simulink model "Trajectory_Tracking_Simulink"  (R2019a)
settings: Solver=VariableStepAuto  StartTime=0.0  StopTime=35  RelTol=1e-3
InitFcn:
  | current_path = pwd;
  | root_folder = strfind(current_path, 'Trajectory_Tracking_Simulation');
  | root_path = current_path( 1 : ( root_folder + 29 ) );
  | initial_folder_path = string(root_path) + '/Initial';
  | addpath(initial_folder_path);
  | run('Initial_Script.m');
model workspace (MAT data in the model file):
  object = [3707764736; 2; 1; 1; 1; 1]
libraries: vrlib x2
settings Model: OrderedModelArguments=off  Creator=Admin  LastModifiedBy=Admin

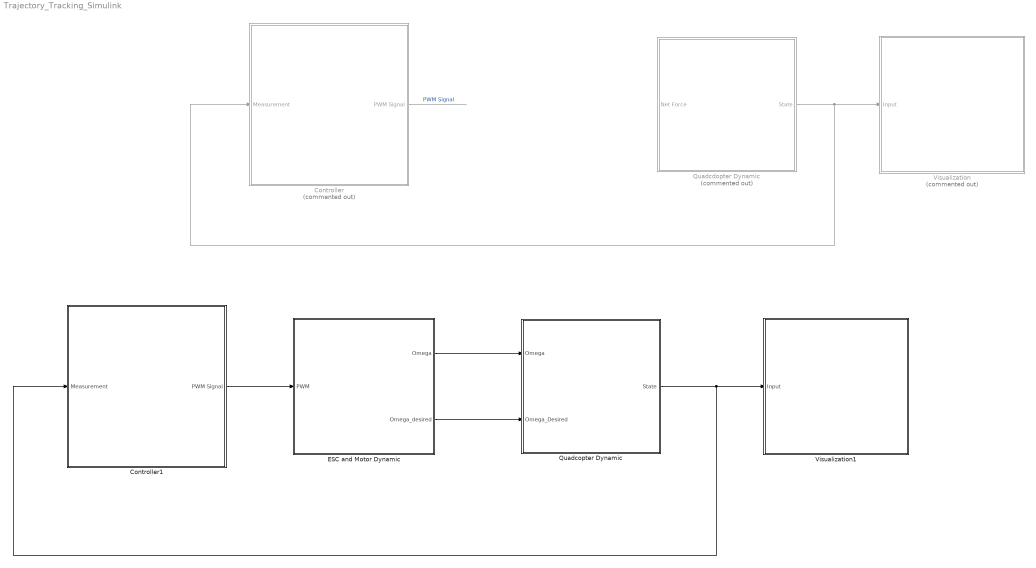
== system Trajectory_Tracking_Simulink ==
  Controller : Subsystem  Commented=on
      mask Display: image('PX4_Picture.jpg');
  Controller1 : Subsystem
      mask Display: image('PX4_Picture.jpg');
  ESC and Motor Dynamic : Subsystem  mask{ct=3.677609694514498e-06, cq=3.677609694514498e-06 / 12, alpha=23 * 1e-3}
      mask prompts: ct "Thrust Coefficent"; cq "Torque Coefficent"; alpha "Delay Time"
      mask DialogControl DescGroupVar Prompt: ESC and Motor Dynamic
      mask DialogControl DescTextVar Prompt: This bock describe ESC and Motor Dynamic
      mask Display: image('ESC_Picture.jpg');
  Quadcdopter Dynamic : Subsystem  Commented=on
      mask Display: image('Kinematic_Diagram.jpg');
  Quadcopter Dynamic : Subsystem
      mask Display: image('Kinematic_Diagram.jpg');
  Visualization : Subsystem  Commented=on
      mask Display: image('VR_Picture.jpg');
  Visualization1 : Subsystem
      mask Display: image('VR_Picture.jpg');
  wires:
  Quadcdopter Dynamic/1("State ") -> Controller/1("Measurement "), Visualization/1("Input ")
  Controller/1(PWM Signal) -> ?  "PWM Signal"
  ? -> Quadcdopter Dynamic/1("Net Force ")  "Force"
  Controller1/1(PWM Signal) -> ESC and Motor Dynamic/1(PWM)
  ESC and Motor Dynamic/1(Omega) -> Quadcopter Dynamic/1("Omega ")
  ESC and Motor Dynamic/2(Omega_desired) -> Quadcopter Dynamic/2(Omega_Desired)
  Quadcopter Dynamic/1("State ") -> Controller1/1("Measurement "), Visualization1/1("Input ")

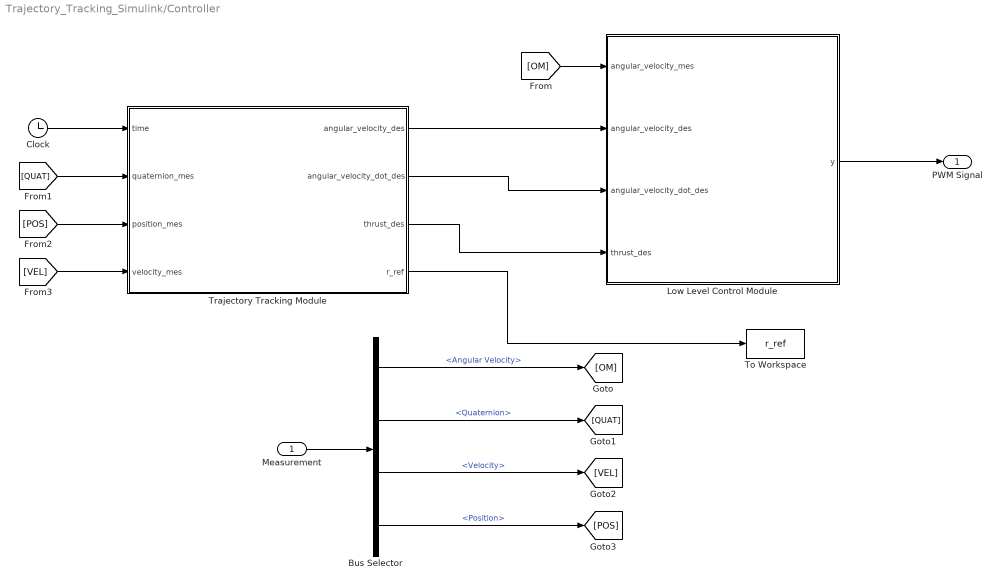
== system Trajectory_Tracking_Simulink/Controller ==
  "Measurement " : Inport
  Bus Selector : BusSelector  OutputSignals=Angular Velocity,Quaternion,Velocity,Position
  Clock : Clock
  Low Level Control Module : MATLAB Function  TreatAsAtomicUnit=on
  To Workspace : ToWorkspace  VariableName=r_ref  SaveFormat=Timeseries  SampleTime=-1
  Trajectory Tracking Module : MATLAB Function  TreatAsAtomicUnit=on
  PWM Signal : Outport
  wires:
  "Measurement "/1 -> Bus Selector/1
  Low Level Control Module/1(y) -> PWM Signal/1
  Bus Selector/1 -> [OM]  "<Angular Velocity>"
  [OM] -> Low Level Control Module/1(angular_velocity_mes)
  Bus Selector/2 -> [QUAT]  "<Quaternion>"
  Bus Selector/3 -> [VEL]  "<Velocity>"
  [QUAT] -> Trajectory Tracking Module/2(quaternion_mes)
  [POS] -> Trajectory Tracking Module/3(position_mes)
  [VEL] -> Trajectory Tracking Module/4(velocity_mes)
  Clock/1 -> Trajectory Tracking Module/1(time)
  Bus Selector/4 -> [POS]  "<Position>"
  Trajectory Tracking Module/1(angular_velocity_des) -> Low Level Control Module/2(angular_velocity_des)
  Trajectory Tracking Module/2(angular_velocity_dot_des) -> Low Level Control Module/3(angular_velocity_dot_des)
  Trajectory Tracking Module/3(thrust_des) -> Low Level Control Module/4(thrust_des)
  Trajectory Tracking Module/4(r_ref) -> To Workspace/1

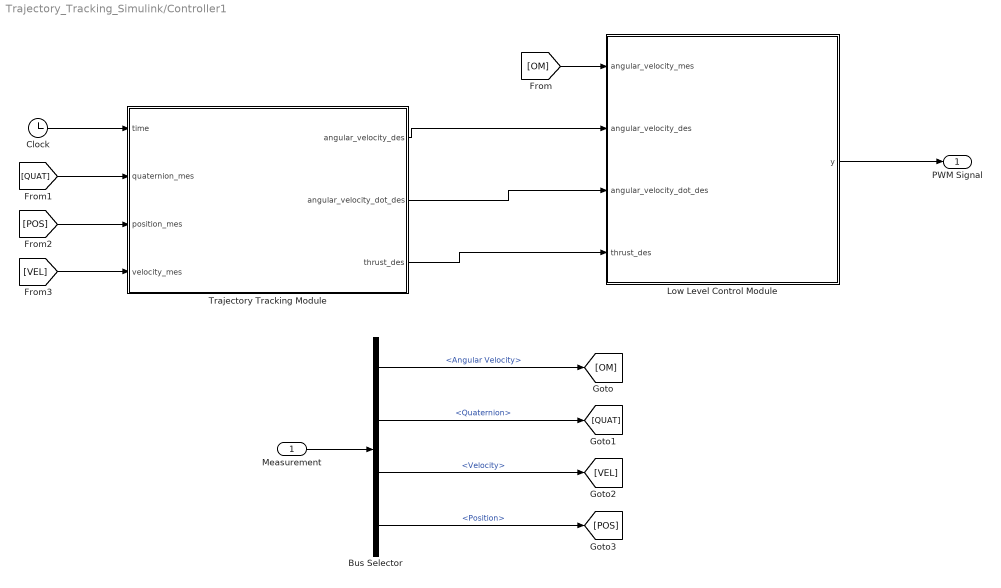
== system Trajectory_Tracking_Simulink/Controller1 ==
  "Measurement " : Inport
  Bus Selector : BusSelector  OutputSignals=Angular Velocity,Quaternion,Velocity,Position
  Clock : Clock
  Low Level Control Module : MATLAB Function  TreatAsAtomicUnit=on
  Trajectory Tracking Module : MATLAB Function  TreatAsAtomicUnit=on
  PWM Signal : Outport
  wires:
  "Measurement "/1 -> Bus Selector/1
  Low Level Control Module/1(y) -> PWM Signal/1
  Bus Selector/1 -> [OM]  "<Angular Velocity>"
  [OM] -> Low Level Control Module/1(angular_velocity_mes)
  Bus Selector/2 -> [QUAT]  "<Quaternion>"
  Bus Selector/3 -> [VEL]  "<Velocity>"
  [QUAT] -> Trajectory Tracking Module/2(quaternion_mes)
  [POS] -> Trajectory Tracking Module/3(position_mes)
  [VEL] -> Trajectory Tracking Module/4(velocity_mes)
  Clock/1 -> Trajectory Tracking Module/1(time)
  Bus Selector/4 -> [POS]  "<Position>"
  Trajectory Tracking Module/1(angular_velocity_des) -> Low Level Control Module/2(angular_velocity_des)
  Trajectory Tracking Module/2(angular_velocity_dot_des) -> Low Level Control Module/3(angular_velocity_dot_des)
  Trajectory Tracking Module/3(thrust_des) -> Low Level Control Module/4(thrust_des)

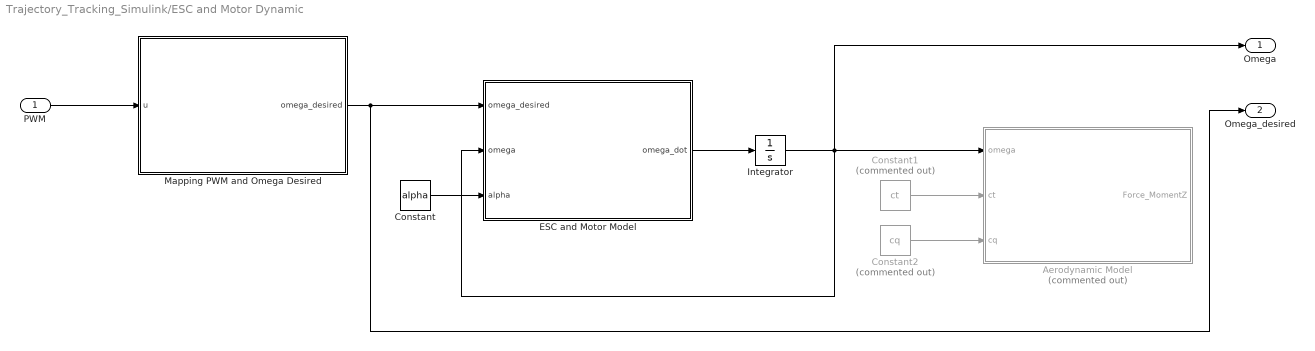
== system Trajectory_Tracking_Simulink/ESC and Motor Dynamic ==
  PWM : Inport
  Aerodynamic Model : MATLAB Function  Commented=on  TreatAsAtomicUnit=on  mask{ct=ct, cq=cq}
      mask prompts: ct "Thrust Coefficent"; cq "Torque Coefficent"
  Constant : Constant  Value=alpha
  Constant1 : Constant  Commented=on  Value=ct
  Constant2 : Constant  Commented=on  Value=cq
  ESC and Motor Model : MATLAB Function  TreatAsAtomicUnit=on  mask{alpha=alpha}
      mask prompts: alpha "Delay Time"
  Integrator : Integrator  InitialCondition=516.5 * ones(4,1)
  Mapping PWM and Omega Desired : MATLAB Function  TreatAsAtomicUnit=on
  Omega : Outport
  Omega_desired : Outport  Port=2
  wires:
  ESC and Motor Model/1(omega_dot) -> Integrator/1
  Integrator/1 -> Omega/1, Aerodynamic Model/1(omega), ESC and Motor Model/2(omega)
  PWM/1 -> Mapping PWM and Omega Desired/1(u)
  Constant/1 -> ESC and Motor Model/3(alpha)
  Constant1/1 -> Aerodynamic Model/2(ct)
  Constant2/1 -> Aerodynamic Model/3(cq)
  Mapping PWM and Omega Desired/1(omega_desired) -> ESC and Motor Model/1(omega_desired), Omega_desired/1

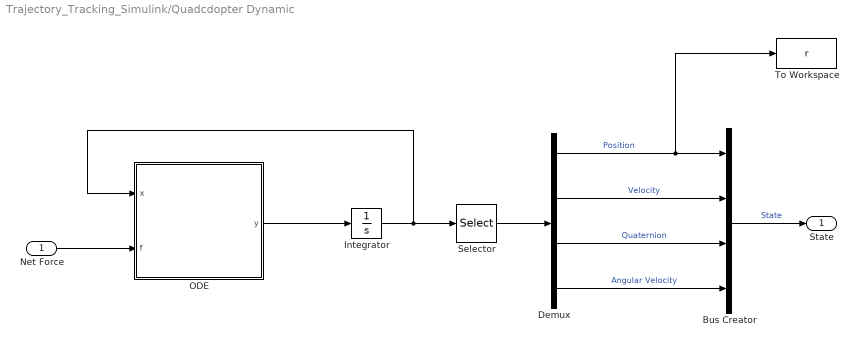
== system Trajectory_Tracking_Simulink/Quadcdopter Dynamic ==
  "Net Force " : Inport
  Bus Creator : BusCreator  Inputs=4
  Demux : Demux  Outputs=[3 3 4 3]
  Integrator : Integrator  InitialCondition=[zeros(3,1); zeros(3,1); [1; 0; 0; 0]; [0; 0; 0]]
  ODE : MATLAB Function  TreatAsAtomicUnit=on
  Selector : Selector  InputPortWidth=13  IndexOptions=Select all  Indices=1  OutputSizes=1
  To Workspace : ToWorkspace  VariableName=r  SaveFormat=Timeseries  SampleTime=-1
  "State " : Outport
  wires:
  Integrator/1 -> Selector/1, ODE/1(x)
  Selector/1 -> Demux/1
  ODE/1(y) -> Integrator/1
  Demux/4 -> Bus Creator/4  "Angular Velocity"
  "Net Force "/1 -> ODE/2(f)
  Demux/1 -> To Workspace/1, Bus Creator/1  "Position"
  Demux/2 -> Bus Creator/2  "Velocity"
  Demux/3 -> Bus Creator/3  "Quaternion"
  Bus Creator/1 -> "State "/1  "State"

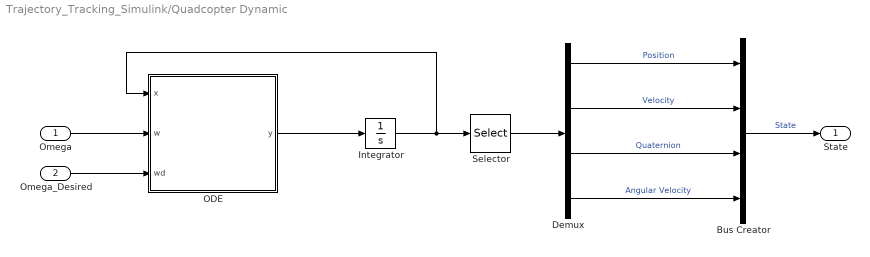
== system Trajectory_Tracking_Simulink/Quadcopter Dynamic ==
  "Omega " : Inport
  Omega_Desired : Inport  Port=2
  Bus Creator : BusCreator  Inputs=4
  Demux : Demux  Outputs=[3 3 4 3]
  Integrator : Integrator  InitialCondition=[zeros(3,1); zeros(3,1); [1; 0;0 ;0]; [0; 0; 0]]
  ODE : MATLAB Function  TreatAsAtomicUnit=on
  Selector : Selector  InputPortWidth=13  IndexOptions=Select all  Indices=1  OutputSizes=1
  "State " : Outport
  wires:
  Integrator/1 -> ODE/1(x), Selector/1
  Selector/1 -> Demux/1
  ODE/1(y) -> Integrator/1
  Demux/4 -> Bus Creator/4  "Angular Velocity"
  "Omega "/1 -> ODE/2(w)
  Demux/1 -> Bus Creator/1  "Position"
  Demux/2 -> Bus Creator/2  "Velocity"
  Demux/3 -> Bus Creator/3  "Quaternion"
  Bus Creator/1 -> "State "/1  "State"
  Omega_Desired/1 -> ODE/3(wd)

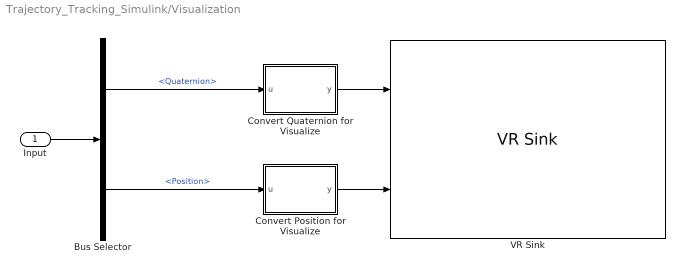
== system Trajectory_Tracking_Simulink/Visualization ==
  "Input " : Inport
  Bus Selector : BusSelector  OutputSignals=Quaternion,Position
  "Convert Position for Visualize " : MATLAB Function  TreatAsAtomicUnit=on
  "Convert Quaternion for Visualize " : MATLAB Function  TreatAsAtomicUnit=on
  VR Sink : vrlib/VR Sink  InstantiateOnLoad=on  SampleTime=0.01  ViewEnable=on  RemoteChange=off  RemoteView=off  FieldsWritten=FBX_Quadcopter_3d_Model_Transform.rotation.4.1.1.double#FBX_Quadcopter_3d_Model_Transform.translation.3.1.1.double  WorldFileName=3d_Model.wrl  AutoView=off  VideoDimensions=[]  AllowVariableSize=off
      settings: SourceProductName=Simulink
  wires:
  "Convert Quaternion for Visualize "/1(y) -> VR Sink/1
  "Convert Position for Visualize "/1(y) -> VR Sink/2
  "Input "/1 -> Bus Selector/1
  Bus Selector/1 -> "Convert Quaternion for Visualize "/1(u)  "<Quaternion>"
  Bus Selector/2 -> "Convert Position for Visualize "/1(u)  "<Position>"

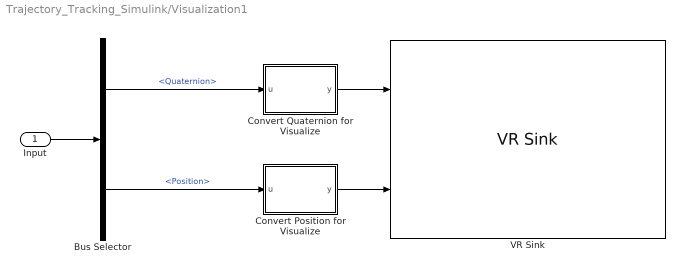
== system Trajectory_Tracking_Simulink/Visualization1 ==
  "Input " : Inport
  Bus Selector : BusSelector  OutputSignals=Quaternion,Position
  "Convert Position for Visualize " : MATLAB Function  TreatAsAtomicUnit=on
  "Convert Quaternion for Visualize " : MATLAB Function  TreatAsAtomicUnit=on
  VR Sink : vrlib/VR Sink  InstantiateOnLoad=on  SampleTime=0.01  ViewEnable=on  RemoteChange=off  RemoteView=off  FieldsWritten=FBX_Quadcopter_3d_Model_Transform.rotation.4.1.1.double#FBX_Quadcopter_3d_Model_Transform.translation.3.1.1.double  WorldFileName=3d_Model.wrl  AutoView=off  VideoDimensions=[]  AllowVariableSize=off  FigureProperties="{'Position', 'Name', 'Viewpoint', 'CameraBound', 'CameraDirection', 'CameraPosition', 'CameraUpVector', 'ZoomFactor', 'Antialiasing', 'Headlight', 'Lighting', 'NavPanel', 'Sound', 'StatusBar', 'Stereo3D', 'Stereo3DCameraOffset', 'Stereo3DHIT', 'ToolBar', 'Textures', 'Transparency', 'Triad', 'Wireframe', 'NavZones', 'NavMode', 'NavSpeed', 'CaptureFileFormat', 'CaptureFileName', 'Record2DCompressMethod', 'Record2DCompressQuality', 'Record2D', 'Record2DFileName', 'Record2DFPS'; [1.0000000000000000e+00   7.6000000000000000e+01   1.9200000000000000e+03   9.5300000000000000e+02], '', 'Perspective View', 'on', [0.0000000000000000e+00   0.0000000000000000e+00  -1.0000000000000000e+00], [0.0000000000000000e+00   0.0000000000000000e+00   0.0000000000000000e+00], [0.0000000000000000e+00   1.0000000000000000e+00   0.0000000000000000e+00], [3.7974983358324148e+00], 'on', 'on', 'on', 'halfbar', 'on', 'on', 'off', [1.0000000149011612e-01], [0.0000000000000000e+00], 'on', 'on', 'on', 'none', 'off', 'off', 'fly', 'normal', 'tif', '%f_anim_%n.tif', 'auto', [7.5000000000000000e+01], 'off', '%f_anim_%n.avi', 'auto'}"
      settings: SourceProductName=Simulink
  wires:
  "Convert Quaternion for Visualize "/1(y) -> VR Sink/1
  "Convert Position for Visualize "/1(y) -> VR Sink/2
  "Input "/1 -> Bus Selector/1
  Bus Selector/1 -> "Convert Quaternion for Visualize "/1(u)  "<Quaternion>"
  Bus Selector/2 -> "Convert Position for Visualize "/1(u)  "<Position>"

== matlab function Trajectory_Tracking_Simulink/Quadcdopter Dynamic/ODE ==
  settings: updateMethod=CONTINUOUS
  data: x input; y output; f input
function y = fcn(x, f)
%%
m = 1.18;
g = [0; 0; -9.81];
a = 0.255/2;
k = 0.0174;
Ixx = 0.0144;
Iyy = 0.0145;
Izz = 0.0156;
J = diag([Ixx, Iyy, Izz]);

%%
r = x(1:3);
v = x(4:6);
q = x(7:10);
omega = x(11:13);

%%
torque = [a, -a, -a, a; -a, -a, a, a; k, -k, k, -k] * f;  
c_body_frame = [0, 0, 0, (1/m) * sum(f)];
c_world_frame = quatmultiply(quatmultiply(q', c_body_frame), quatconj(q'))';
OMEGA = 0.5 * [0, -omega'; omega, -skew(omega)];
x_dot = zeros(13,1);
x_dot(1:3) = v;
x_dot(4:6) = g + c_world_frame(2:end);
x_dot(7:10) = OMEGA * q;
x_dot(11:13) = J \ (torque - cross(omega, J * omega));

%%
y = x_dot;
end

== matlab function Trajectory_Tracking_Simulink/Controller/Low Level Control Module ==
  settings: updateMethod=DISCRETE  sampleTime=1/200
  data: angular_velocity_mes input; angular_velocity_des input; y output; angular_velocity_dot_des input; thrust_des input
function y = fcn(angular_velocity_mes, angular_velocity_des, angular_velocity_dot_des, thrust_des)
    persistent mixer omega_controller
    if isempty(mixer) 
        mixer = Mixer();
    end
    
    if isempty(omega_controller)
        omega_controller = AngularVelocityController();
    end
    
    omega_controller.updateAngularVelocityDesired(angular_velocity_des, angular_velocity_dot_des);
    omega_controller.updateTorqueDesired(angular_velocity_mes);
    
    
    mixer.setThrustTorqueSetpoint(omega_controller.torque_des, thrust_des);
    mixer.computeControlSignal();
    
    y = mixer.control_signal;
end

== matlab function Trajectory_Tracking_Simulink/Quadcopter Dynamic/ODE ==
  settings: updateMethod=CONTINUOUS
  data: x input; y output; w input; wd input
function y = fcn(x, w, wd)
%%
m = 1.18; % vehicle's mass
g = [0; 0; -9.81]; % gravity vector
a = 0.255/2; % half arm lenght
Ixx = 0.0257; % 
Iyy = 0.0255; %
Izz = 0.0321; %
Io = diag([Ixx, Iyy, Izz]); % vehicle's moment inertia
Ir = 8.67 * 1e-5; % rotor blade moment inertial
ct = 3.677609694514498e-06; % thrust coefficent
cq = ct / 12; % moment coefficient
rc = [7 * 1e-2; 6 * 1e-2; 0]; % center of mass in body frame
rc = [0;0;0];
alpha = 23 * 1e-3; % time delay of ESC + MOTOR + BLADE
%%
r = x(1:3);
v = x(4:6);
q = x(7:10);
W = x(11:13);

%% 
r_dot = v;

q_dot = 0.5 * quatmultiply( q', [0, W'] )';

G = [a*ct, -a*ct,  -a*ct, a*ct;
    -a*ct,  -a*ct, a*ct,  a*ct;
       cq,   -cq,    cq,   -cq;];
C0 = ct * skew(rc) * [zeros(2,4); ones(1,4)];
C1 = (1/alpha) * [zeros(2,4); -1, 1, -1, 1];
C2 = [0, 1, 0; -1, 0, 0; 0, 0, 0];
C3 = [-1 1 -1 1];
tau_g = Ir * ( C1 * (wd - w) + C2 * W * C3 * w );
tau_g = [0;0;0];
W_dot = (Io + m * skew(rc) * skew(rc)) \ ( (G - C0) * w.^2 - tau_g - cross( W, ( Io + m * (rc * rc')) * W ) );

Rz = [2 * (q(1) * q(3) + q(2) * q(4)); 2 * (q(3) * q(4) - q(1) * q(2)); 2 * (q(1)^2 +  q(4)^2) - 1] ;
F = m * g +  ct * Rz * [1 1 1 1] * w.^2;
term_1 = quatmultiply(quatmultiply(q', [0, cross(W_dot, rc)']), quatconj(q'));
term_2 = quatmultiply(quatmultiply(q', [0, (W' * W) * rc']), quatconj(q'));
v_dot = F/m - term_1(2:end)' + term_2(2:end)';

%%
x_dot = [r_dot; 
         v_dot; 
         q_dot;
         W_dot];
%%
y = x_dot;
end

== matlab function Trajectory_Tracking_Simulink/Visualization/Convert Position for Visualize  ==
  data: u input; y output
function y = fcn(u)
temp = quatmultiply(quatmultiply([0.5, -0.5, 0.5, 0.5], [0, u']), [0.5, 0.5, -0.5, -0.5]);
y = temp(2:end);

== matlab function Trajectory_Tracking_Simulink/Visualization/Convert Quaternion for Visualize  ==
  data: u input; y output
function y = fcn(u)
u = u./norm(u);
rotation_angle = 2 * acos(u(1));
rotation_axis = u(2:end)./(sin(0.5 * rotation_angle));
y = [0, -1, 0, 0; 0, 0, 1, 0; -1, 0, 0, 0; 0, 0, 0, 1]*[rotation_axis; rotation_angle];

== matlab function Trajectory_Tracking_Simulink/Controller/Trajectory Tracking Module ==
  settings: updateMethod=DISCRETE  sampleTime=1/50
  data: time input; quaternion_mes input; position_mes input; angular_velocity_des output; angular_velocity_dot_des output; thrust_des output; velocity_mes input; r_ref output
function [angular_velocity_des, angular_velocity_dot_des, thrust_des, r_ref] = fcn(time, quaternion_mes, position_mes, velocity_mes)
    persistent observer position_controller attitude_controller generator
    if isempty(observer)
        observer = GeneralObserver();
        observer.getInitMeasurement(quaternion_mes, position_mes);
        observer.init_time = time;
    end
    
    if isempty(position_controller)
        position_controller = PositionController();
    end
    
    if isempty(attitude_controller)
        attitude_controller = AttitudeController();
    end    
    
    if isempty(generator)
        generator = TrajectoryGenerator();
    end      

 
    observer.adjustMeasurement(quaternion_mes, position_mes, velocity_mes);
    observer.current_time = time;
    generator.updateTrajectorieStates(observer);
    
    position_controller.updateAcceleration(generator, observer);
    observer.computeQuadError(position_controller.acceleration_des, generator.phi);
	position_controller.updateAngularRef(generator , observer);

	attitude_controller.updateAngularVelocityDesired(observer, position_controller);
    
    angular_velocity_des = attitude_controller.omega_des;
    angular_velocity_dot_des = position_controller.omega_dot_ref;
    thrust_des = observer.c_des;
    
    r_ref = generator.r_ref;
    
end

== matlab function Trajectory_Tracking_Simulink/ESC and Motor Dynamic/Aerodynamic Model ==
  settings: updateMethod=CONTINUOUS
  data: omega input; Force_MomentZ output; ct input; cq input
function Force_MomentZ = fcn(omega, ct, cq)
% ct = 3.677609694514498e-06;
% cq = ct / 1.5;
Force_MomentZ = [ct * omega.^2; cq * omega.^2];           
end

== matlab function Trajectory_Tracking_Simulink/ESC and Motor Dynamic/ESC and Motor Model ==
  settings: updateMethod=CONTINUOUS
  data: omega_desired input; omega_dot output; omega input; alpha input
function omega_dot = fcn(omega_desired, omega, alpha)
% alpha = 23 * 1e-3;
omega_dot = (1 / alpha) * (omega_desired - omega);             
end

== matlab function Trajectory_Tracking_Simulink/ESC and Motor Dynamic/Mapping PWM and Omega Desired ==
  settings: updateMethod=CONTINUOUS
  data: u input; omega_desired output
function omega_desired = fcn(u)
omega_d_max = 1701;
omega_d_min = 516.5;
omega_desired = (omega_d_max - omega_d_min) * u + omega_d_min;
end

== matlab function Trajectory_Tracking_Simulink/Visualization1/Convert Position for Visualize  ==
  data: u input; y output
function y = fcn(u)
temp = quatmultiply(quatmultiply([0.5, -0.5, 0.5, 0.5], [0, u']), [0.5, 0.5, -0.5, -0.5]);
y = temp(2:end);

== matlab function Trajectory_Tracking_Simulink/Visualization1/Convert Quaternion for Visualize  ==
  data: u input; y output
function y = fcn(u)
u = u./norm(u);
rotation_angle = 2 * acos(u(1));
rotation_axis = u(2:end)./(sin(0.5 * rotation_angle));
y = [0, -1, 0, 0; 0, 0, 1, 0; -1, 0, 0, 0; 0, 0, 0, 1]*[rotation_axis; rotation_angle];

== matlab function Trajectory_Tracking_Simulink/Controller1/Low Level Control Module ==
  settings: updateMethod=DISCRETE  sampleTime=1/200
  data: angular_velocity_mes input; angular_velocity_des input; y output; angular_velocity_dot_des input; thrust_des input
function y = fcn(angular_velocity_mes, angular_velocity_des, angular_velocity_dot_des, thrust_des)
    persistent mixer omega_controller
    if isempty(mixer) 
        mixer = Mixer();
    end
    
    if isempty(omega_controller)
        omega_controller = AngularVelocityController();
    end
    
    omega_controller.updateAngularVelocityDesired(angular_velocity_des, angular_velocity_dot_des);
    omega_controller.updateTorqueDesired(angular_velocity_mes);
    
    
    mixer.setThrustTorqueSetpoint(omega_controller.torque_des, thrust_des);
    mixer.computeControlSignal();
    
    y = mixer.control_signal;
end

== matlab function Trajectory_Tracking_Simulink/Controller1/Trajectory Tracking Module ==
  settings: updateMethod=DISCRETE  sampleTime=1/50
  data: time input; quaternion_mes input; position_mes input; angular_velocity_des output; angular_velocity_dot_des output; thrust_des output; velocity_mes input
function [angular_velocity_des, angular_velocity_dot_des, thrust_des] = fcn(time, quaternion_mes, position_mes, velocity_mes)
    persistent observer position_controller attitude_controller generator
    if isempty(observer)
        observer = GeneralObserver();
        observer.getInitMeasurement(quaternion_mes, position_mes);
        observer.init_time = time;
    end
    
    if isempty(position_controller)
        position_controller = PositionController();
    end
    
    if isempty(attitude_controller)
        attitude_controller = AttitudeController();
    end    
    
    if isempty(generator)
        generator = TrajectoryGenerator();
    end      

 
    observer.adjustMeasurement(quaternion_mes, position_mes, velocity_mes);
    observer.current_time = time;
    generator.updateTrajectorieStates(observer);
    
    position_controller.updateAcceleration(generator, observer);
    observer.computeQuadError(position_controller.acceleration_des, generator.phi);
	position_controller.updateAngularRef(generator , observer);

	attitude_controller.updateAngularVelocityDesired(observer, position_controller);
    
    angular_velocity_des = attitude_controller.omega_des;
    angular_velocity_dot_des = position_controller.omega_dot_ref;
    thrust_des = observer.c_des;
    
    
end
